simulink model "doc_filterdelay"  (Simulink 6.0)
settings: Solver=ode45  StartTime=0.0  StopTime=5  RelTol=1e-3
undefined symbols (not defined in the file): slcm
libraries: commanapbnd2 x2, dspsrcs4 x1
settings Model: Creator=agaltman  LastModifiedBy=agaltman  ProdHWDeviceType=Specified
settings DataIOCC: SignalLoggingName=logsOut
settings OptimizationCC: BlockReduction=off  BooleanDataType=off  MultiInstanced=off
settings FormatCC: IgnoreBidirectionalLines=off
settings HardwareCC: ProdHWDeviceType=Specified
settings CodeAppCC: FileBanners=off  CustomSymbols=off  MangleLength=5
settings GRTTargetCC: TargetFcnLib=iso_c_tmw.mat  IsERTTarget=off

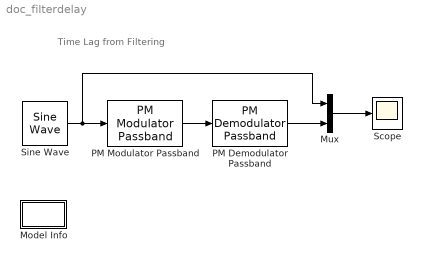
== system doc_filterdelay ==
  note: Time Lag from Filtering
  Model Info : Subsystem  LoadFcn=slcm LoadBlock;  InitFcn=slcm('UpdateAllCMBlocksInThisModelInit')  mask(CMBlock){InitialSaveTempField=, InitialBlockCM=none, BlockCM=none, Frame=on, SaveTempField=, DisplayStringWithTags=Info, MaskDisplayString=Info, HorizontalTextAlignment=Center, LeftAlignmentValue=0.5, SourceBlockDiagram=doc_filterdelay, TagMaxNumber=20, CMTag1=, CMTag2=, CMTag3=, CMTag4=, CMTag5=, CMTag6=, CMTag7=, CMTag8=, CMTag9=, CMTag10=, CMTag11=, CMTag12=, CMTag13=, CMTag14=, CMTag15=, CMTag16=, CMTag17=, CMTag18=, CMTag19=, CMTag20=}
      mask help: This block allows revision control information to be displayed within the model.
      settings: CopyFcn=slcm CopyBlock;  DeleteFcn=slcm Cancel;  PostSaveFcn=slcm('UpdateAllCMBlocksInThisModel')  NameChangeFcn=slcm Rename;  OpenFcn=commdemohelp;
      mask Display: text(str2num(LeftAlignmentValue), 0.5, MaskDisplayString, 'HorizontalAlignment', HorizontalTextAlignment)
  Mux : Mux  Inputs=2
  PM Demodulator Passband : commanapbnd2/PM Demodulator Passband  Fc=100  Ph=0  Kc=1  num=[4.57 9.14 4.57]*.01  den=[1 -1.3108 .4936]  HzPerVolt=1  ts=0.001
  PM Modulator Passband : commanapbnd2/PM Modulator Passband  Fc=100  Ph=0  Kc=1  td=Inf
  Scope : Scope
  Sine Wave : dspsrcs4/Sine Wave  Amplitude=1  Frequency=1  Phase=0  SampleMode=Discrete  OutComplex=Real  CompMethod=Trigonometric fcn  TableSize=Speed  SampleTime=1/1000  SamplesPerFrame=1  dataType=double  wordLen=16  udDataType=sfix(16)  fracBitsMode=Best precision  numFracBits=14  ResetState=Restart at time zero
  wires:
  Sine Wave/1 -> Mux/1, PM Modulator Passband/1
  PM Modulator Passband/1 -> PM Demodulator Passband/1
  PM Demodulator Passband/1 -> Mux/2
  Mux/1 -> Scope/1

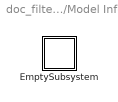
== system doc_filterdelay/Model Info ==
  EmptySubsystem : Subsystem

== system doc_filterdelay/Model Info/EmptySubsystem ==
